simulink library "SIXOSEM_F_STAGE_MASTER_backup20190220"  (Simulink 8.6)
settings: Solver=ode45  StartTime=0.0  StopTime=10.0  RelTol=1e-3
libraries: cdsEpicsOut x52, cdsFilt x31, cdsTP x24, cdsFiltCtrl x9, cdsEpicsIn x9, cdsMuxMatrix x6, VIS_LIB x3, cdsEpicsBinIn x2, lockin x2, SIXOSEM_F_COILOUTF_MASTER x1, rtdemod x1, cdsOsc x1
(part 4 of 5)

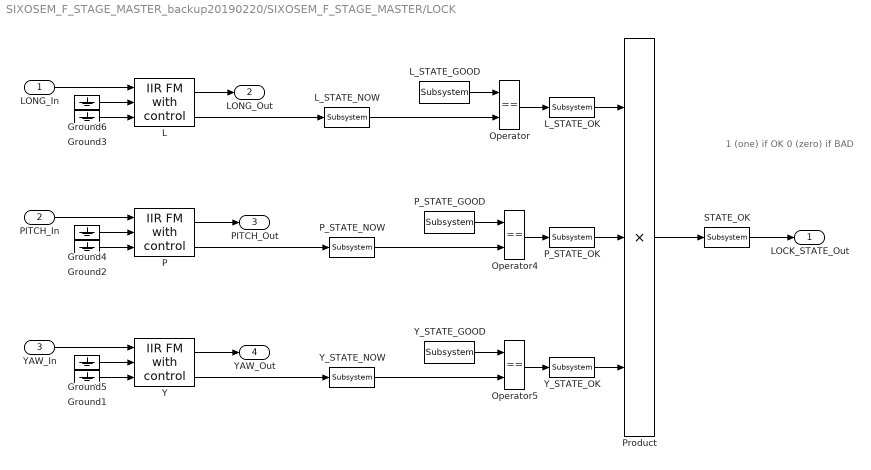
== system SIXOSEM_F_STAGE_MASTER_backup20190220/SIXOSEM_F_STAGE_MASTER/LOCK ==
  note: 1 (one) if OK
      | 0 (zero) if BAD
  LONG_In : Inport
  PITCH_In : Inport  Port=2
  YAW_In : Inport  Port=3
  Ground{1..6} (6 alike) : Ground
  L : cdsFiltCtrl/IIR FM with control  Tag=cdsFiltCtrl  Description=|
      | cdsFiltCntrl is the standard IIR filter module (exactly the same as cdsFilt) but with added control data output 'Ctrl'. Filter module digital signal output appears on the first output, which is called 'Val'. 'Ctrl' output has a bit pattern encoding the state of filter's on/off switches (FM1 through FM10). The bit values are:
      |                                                                                                                                                                                                                                                                                                                                       
      | module 	hex	dec                                                                                                                                                                                                                                                                                                                       
      | -----------------------                                                                                                                                                                                                                                                                                                               
      | FM1	0x20                    32                                                                                                                                                                                                                                                                                                        
      | FM2	0x80                     128                                                                                                                                                                                                                                                                                                      
      | FM3	0x200                   512                                                                                                                                                                                                                                                                                                       
      | FM4	0x800                   2048                                                                                                                                                                                                                                                                                                      
      | FM5	0x2000                 8192                                                                                                                                                                                                                                                                                                       
      | FM6	0x8000                 32768                                                                                                                                                                                                                                                                                                      
      | FM7	0x20000                131072                                                                                                                                                                                                                                                                                                     
      | FM8	0x80000                 524288                                                                                                                                                                                                                                                                                                    
      | FM9	0x200000               2097152                                                                                                                                                                                                                                                                                                    
      | FM10	0x800000               8388608                                                                                                                                                                                                                                                                                                   
      |                                                                                                                                                                                                                                                                                                                                       
      | This bit data can be used to drive some other switches or it can be output using a binary I/O module.
      settings: AttributesFormatString=%<Tag>
  L_STATE_GOOD : cdsEpicsIn/Subsystem  Tag=cdsEpicsIn  Description=|
      | Purpose:                                                                              
      | Create an EPICS input channel connection to the FE realtime controls.                 
      |                                                                                       
      | Operation:                                                                            
      | Outputs value from an EPICS ai record. Value is floating point with a precision of 3..
      |                                                                                       
      | Usage:                                                                                
      | Name the part with the desired EPICS channel name.
      settings: AttributesFormatString=%<Tag>
  L_STATE_NOW : cdsEpicsOut/Subsystem  Tag=cdsEpicsOutput  Description=|
      | Purpose:                                          
      | Output a FE signal to an EPICS channel.           
      |                                                   
      | Operation:                                        
      | Takes input value and passes it to EPICS record.  
      |                                                   
      | Usage:                                            
      | Name the part with the desired EPICS rrecord name.
      settings: AttributesFormatString=%<Tag>
  L_STATE_OK : cdsEpicsOut/Subsystem  Tag=cdsEpicsOutput  Description=|
      | Purpose:                                          
      | Output a FE signal to an EPICS channel.           
      |                                                   
      | Operation:                                        
      | Takes input value and passes it to EPICS record.  
      |                                                   
      | Usage:                                            
      | Name the part with the desired EPICS rrecord name.
      settings: AttributesFormatString=%<Tag>
  Operator : RelationalOperator  Operator===  OutDataTypeStr=boolean
  Operator4 : RelationalOperator  Operator===  OutDataTypeStr=boolean
  Operator5 : RelationalOperator  Operator===  OutDataTypeStr=boolean
  P : cdsFiltCtrl/IIR FM with control  Tag=cdsFiltCtrl  Description=|
      | cdsFiltCntrl is the standard IIR filter module (exactly the same as cdsFilt) but with added control data output 'Ctrl'. Filter module digital signal output appears on the first output, which is called 'Val'. 'Ctrl' output has a bit pattern encoding the state of filter's on/off switches (FM1 through FM10). The bit values are:
      |                                                                                                                                                                                                                                                                                                                                       
      | module 	hex	dec                                                                                                                                                                                                                                                                                                                       
      | -----------------------                                                                                                                                                                                                                                                                                                               
      | FM1	0x20                    32                                                                                                                                                                                                                                                                                                        
      | FM2	0x80                     128                                                                                                                                                                                                                                                                                                      
      | FM3	0x200                   512                                                                                                                                                                                                                                                                                                       
      | FM4	0x800                   2048                                                                                                                                                                                                                                                                                                      
      | FM5	0x2000                 8192                                                                                                                                                                                                                                                                                                       
      | FM6	0x8000                 32768                                                                                                                                                                                                                                                                                                      
      | FM7	0x20000                131072                                                                                                                                                                                                                                                                                                     
      | FM8	0x80000                 524288                                                                                                                                                                                                                                                                                                    
      | FM9	0x200000               2097152                                                                                                                                                                                                                                                                                                    
      | FM10	0x800000               8388608                                                                                                                                                                                                                                                                                                   
      |                                                                                                                                                                                                                                                                                                                                       
      | This bit data can be used to drive some other switches or it can be output using a binary I/O module.
      settings: AttributesFormatString=%<Tag>
  P_STATE_GOOD : cdsEpicsIn/Subsystem  Tag=cdsEpicsIn  Description=|
      | Purpose:                                                                              
      | Create an EPICS input channel connection to the FE realtime controls.                 
      |                                                                                       
      | Operation:                                                                            
      | Outputs value from an EPICS ai record. Value is floating point with a precision of 3..
      |                                                                                       
      | Usage:                                                                                
      | Name the part with the desired EPICS channel name.
      settings: AttributesFormatString=%<Tag>
  P_STATE_NOW : cdsEpicsOut/Subsystem  Tag=cdsEpicsOutput  Description=|
      | Purpose:                                          
      | Output a FE signal to an EPICS channel.           
      |                                                   
      | Operation:                                        
      | Takes input value and passes it to EPICS record.  
      |                                                   
      | Usage:                                            
      | Name the part with the desired EPICS rrecord name.
      settings: AttributesFormatString=%<Tag>
  P_STATE_OK : cdsEpicsOut/Subsystem  Tag=cdsEpicsOutput  Description=|
      | Purpose:                                          
      | Output a FE signal to an EPICS channel.           
      |                                                   
      | Operation:                                        
      | Takes input value and passes it to EPICS record.  
      |                                                   
      | Usage:                                            
      | Name the part with the desired EPICS rrecord name.
      settings: AttributesFormatString=%<Tag>
  Product : Product  Inputs=3  RndMeth=Zero
  STATE_OK : cdsEpicsOut/Subsystem  Tag=cdsEpicsOutput  Description=|
      | Purpose:                                          
      | Output a FE signal to an EPICS channel.           
      |                                                   
      | Operation:                                        
      | Takes input value and passes it to EPICS record.  
      |                                                   
      | Usage:                                            
      | Name the part with the desired EPICS rrecord name.
      settings: AttributesFormatString=%<Tag>
  Y : cdsFiltCtrl/IIR FM with control  Tag=cdsFiltCtrl  Description=|
      | cdsFiltCntrl is the standard IIR filter module (exactly the same as cdsFilt) but with added control data output 'Ctrl'. Filter module digital signal output appears on the first output, which is called 'Val'. 'Ctrl' output has a bit pattern encoding the state of filter's on/off switches (FM1 through FM10). The bit values are:
      |                                                                                                                                                                                                                                                                                                                                       
      | module 	hex	dec                                                                                                                                                                                                                                                                                                                       
      | -----------------------                                                                                                                                                                                                                                                                                                               
      | FM1	0x20                    32                                                                                                                                                                                                                                                                                                        
      | FM2	0x80                     128                                                                                                                                                                                                                                                                                                      
      | FM3	0x200                   512                                                                                                                                                                                                                                                                                                       
      | FM4	0x800                   2048                                                                                                                                                                                                                                                                                                      
      | FM5	0x2000                 8192                                                                                                                                                                                                                                                                                                       
      | FM6	0x8000                 32768                                                                                                                                                                                                                                                                                                      
      | FM7	0x20000                131072                                                                                                                                                                                                                                                                                                     
      | FM8	0x80000                 524288                                                                                                                                                                                                                                                                                                    
      | FM9	0x200000               2097152                                                                                                                                                                                                                                                                                                    
      | FM10	0x800000               8388608                                                                                                                                                                                                                                                                                                   
      |                                                                                                                                                                                                                                                                                                                                       
      | This bit data can be used to drive some other switches or it can be output using a binary I/O module.
      settings: AttributesFormatString=%<Tag>
  Y_STATE_GOOD : cdsEpicsIn/Subsystem  Tag=cdsEpicsIn  Description=|
      | Purpose:                                                                              
      | Create an EPICS input channel connection to the FE realtime controls.                 
      |                                                                                       
      | Operation:                                                                            
      | Outputs value from an EPICS ai record. Value is floating point with a precision of 3..
      |                                                                                       
      | Usage:                                                                                
      | Name the part with the desired EPICS channel name.
      settings: AttributesFormatString=%<Tag>
  Y_STATE_NOW : cdsEpicsOut/Subsystem  Tag=cdsEpicsOutput  Description=|
      | Purpose:                                          
      | Output a FE signal to an EPICS channel.           
      |                                                   
      | Operation:                                        
      | Takes input value and passes it to EPICS record.  
      |                                                   
      | Usage:                                            
      | Name the part with the desired EPICS rrecord name.
      settings: AttributesFormatString=%<Tag>
  Y_STATE_OK : cdsEpicsOut/Subsystem  Tag=cdsEpicsOutput  Description=|
      | Purpose:                                          
      | Output a FE signal to an EPICS channel.           
      |                                                   
      | Operation:                                        
      | Takes input value and passes it to EPICS record.  
      |                                                   
      | Usage:                                            
      | Name the part with the desired EPICS rrecord name.
      settings: AttributesFormatString=%<Tag>
  LOCK_STATE_Out : Outport
  LONG_Out : Outport  Port=2
  PITCH_Out : Outport  Port=3
  YAW_Out : Outport  Port=4
  wires:
  Ground6/1 -> L/2
  L_STATE_GOOD/1 -> Operator/1
  L/2 -> L_STATE_NOW/1
  L/1 -> LONG_Out/1
  LONG_In/1 -> L/1
  P/1 -> PITCH_Out/1
  Ground4/1 -> P/2
  PITCH_In/1 -> P/1
  P_STATE_GOOD/1 -> Operator4/1
  P/2 -> P_STATE_NOW/1
  Ground5/1 -> Y/2
  YAW_In/1 -> Y/1
  Y_STATE_GOOD/1 -> Operator5/1
  Y/2 -> Y_STATE_NOW/1
  Y/1 -> YAW_Out/1
  Operator/1 -> L_STATE_OK/1
  Operator4/1 -> P_STATE_OK/1
  Operator5/1 -> Y_STATE_OK/1
  Product/1 -> STATE_OK/1
  P_STATE_OK/1 -> Product/2
  L_STATE_OK/1 -> Product/1
  Y_STATE_OK/1 -> Product/3
  STATE_OK/1 -> LOCK_STATE_Out/1
  L_STATE_NOW/1 -> Operator/2
  Y_STATE_NOW/1 -> Operator5/2
  P_STATE_NOW/1 -> Operator4/2
  Ground1/1 -> Y/3
  Ground2/1 -> P/3
  Ground3/1 -> L/3

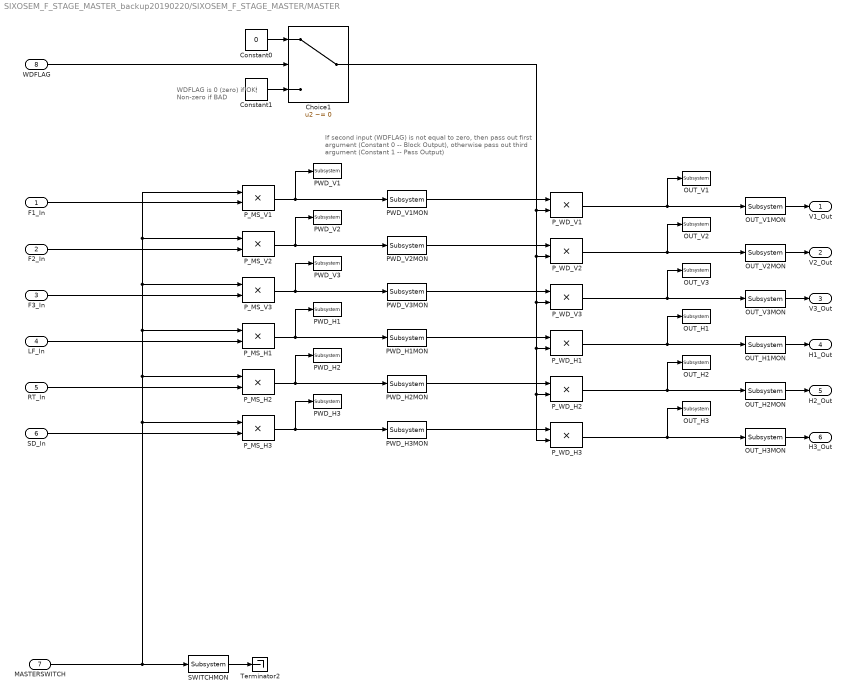
== system SIXOSEM_F_STAGE_MASTER_backup20190220/SIXOSEM_F_STAGE_MASTER/MASTER ==
  note: WDFLAG is 0 (zero) if OK,
      | Non-zero if BAD
  note: If second input (WDFLAG) is not equal to zero,
      | then pass out first argument (Constant 0 -- Block Output),
      | otherwise pass out third argument (Constant 1 -- Pass Output)
  F1_In : Inport
  F2_In : Inport  Port=2
  F3_In : Inport  Port=3
  LF_In : Inport  Port=4
  RT_In : Inport  Port=5
  SD_In : Inport  Port=6
  MASTERSWITCH : Inport  Port=7
  WDFLAG : Inport  Port=8
  Choice1 : Switch  Criteria=u2 ~= 0  Threshold=0.5
  Constant0 : Constant  Value=0
  Constant1 : Constant
  OUT_H1 : cdsTP/Subsystem  Tag=Test Point
      settings: AttributesFormatString=%<Tag>
  OUT_H1MON : cdsEpicsOut/Subsystem  Tag=cdsEpicsOutput  Description=|
      | Purpose:                                          
      | Output a FE signal to an EPICS channel.           
      |                                                   
      | Operation:                                        
      | Takes input value and passes it to EPICS record.  
      |                                                   
      | Usage:                                            
      | Name the part with the desired EPICS rrecord name.
      settings: AttributesFormatString=%<Tag>
  OUT_H2 : cdsTP/Subsystem  Tag=Test Point
      settings: AttributesFormatString=%<Tag>
  OUT_H2MON : cdsEpicsOut/Subsystem  Tag=cdsEpicsOutput  Description=|
      | Purpose:                                          
      | Output a FE signal to an EPICS channel.           
      |                                                   
      | Operation:                                        
      | Takes input value and passes it to EPICS record.  
      |                                                   
      | Usage:                                            
      | Name the part with the desired EPICS rrecord name.
      settings: AttributesFormatString=%<Tag>
  OUT_H3 : cdsTP/Subsystem  Tag=Test Point
      settings: AttributesFormatString=%<Tag>
  OUT_H3MON : cdsEpicsOut/Subsystem  Tag=cdsEpicsOutput  Description=|
      | Purpose:                                          
      | Output a FE signal to an EPICS channel.           
      |                                                   
      | Operation:                                        
      | Takes input value and passes it to EPICS record.  
      |                                                   
      | Usage:                                            
      | Name the part with the desired EPICS rrecord name.
      settings: AttributesFormatString=%<Tag>
  OUT_V1 : cdsTP/Subsystem  Tag=Test Point
      settings: AttributesFormatString=%<Tag>
  OUT_V1MON : cdsEpicsOut/Subsystem  Tag=cdsEpicsOutput  Description=|
      | Purpose:                                          
      | Output a FE signal to an EPICS channel.           
      |                                                   
      | Operation:                                        
      | Takes input value and passes it to EPICS record.  
      |                                                   
      | Usage:                                            
      | Name the part with the desired EPICS rrecord name.
      settings: AttributesFormatString=%<Tag>
  OUT_V2 : cdsTP/Subsystem  Tag=Test Point
      settings: AttributesFormatString=%<Tag>
  OUT_V2MON : cdsEpicsOut/Subsystem  Tag=cdsEpicsOutput  Description=|
      | Purpose:                                          
      | Output a FE signal to an EPICS channel.           
      |                                                   
      | Operation:                                        
      | Takes input value and passes it to EPICS record.  
      |                                                   
      | Usage:                                            
      | Name the part with the desired EPICS rrecord name.
      settings: AttributesFormatString=%<Tag>
  OUT_V3 : cdsTP/Subsystem  Tag=Test Point
      settings: AttributesFormatString=%<Tag>
  OUT_V3MON : cdsEpicsOut/Subsystem  Tag=cdsEpicsOutput  Description=|
      | Purpose:                                          
      | Output a FE signal to an EPICS channel.           
      |                                                   
      | Operation:                                        
      | Takes input value and passes it to EPICS record.  
      |                                                   
      | Usage:                                            
      | Name the part with the desired EPICS rrecord name.
      settings: AttributesFormatString=%<Tag>
  PWD_H1 : cdsTP/Subsystem  Tag=Test Point
      settings: AttributesFormatString=%<Tag>
  PWD_H1MON : cdsEpicsOut/Subsystem  Tag=cdsEpicsOutput  Description=|
      | Purpose:                                          
      | Output a FE signal to an EPICS channel.           
      |                                                   
      | Operation:                                        
      | Takes input value and passes it to EPICS record.  
      |                                                   
      | Usage:                                            
      | Name the part with the desired EPICS rrecord name.
      settings: AttributesFormatString=%<Tag>
  PWD_H2 : cdsTP/Subsystem  Tag=Test Point
      settings: AttributesFormatString=%<Tag>
  PWD_H2MON : cdsEpicsOut/Subsystem  Tag=cdsEpicsOutput  Description=|
      | Purpose:                                          
      | Output a FE signal to an EPICS channel.           
      |                                                   
      | Operation:                                        
      | Takes input value and passes it to EPICS record.  
      |                                                   
      | Usage:                                            
      | Name the part with the desired EPICS rrecord name.
      settings: AttributesFormatString=%<Tag>
  PWD_H3 : cdsTP/Subsystem  Tag=Test Point
      settings: AttributesFormatString=%<Tag>
  PWD_H3MON : cdsEpicsOut/Subsystem  Tag=cdsEpicsOutput  Description=|
      | Purpose:                                          
      | Output a FE signal to an EPICS channel.           
      |                                                   
      | Operation:                                        
      | Takes input value and passes it to EPICS record.  
      |                                                   
      | Usage:                                            
      | Name the part with the desired EPICS rrecord name.
      settings: AttributesFormatString=%<Tag>
  PWD_V1 : cdsTP/Subsystem  Tag=Test Point
      settings: AttributesFormatString=%<Tag>
  PWD_V1MON : cdsEpicsOut/Subsystem  Tag=cdsEpicsOutput  Description=|
      | Purpose:                                          
      | Output a FE signal to an EPICS channel.           
      |                                                   
      | Operation:                                        
      | Takes input value and passes it to EPICS record.  
      |                                                   
      | Usage:                                            
      | Name the part with the desired EPICS rrecord name.
      settings: AttributesFormatString=%<Tag>
  PWD_V2 : cdsTP/Subsystem  Tag=Test Point
      settings: AttributesFormatString=%<Tag>
  PWD_V2MON : cdsEpicsOut/Subsystem  Tag=cdsEpicsOutput  Description=|
      | Purpose:                                          
      | Output a FE signal to an EPICS channel.           
      |                                                   
      | Operation:                                        
      | Takes input value and passes it to EPICS record.  
      |                                                   
      | Usage:                                            
      | Name the part with the desired EPICS rrecord name.
      settings: AttributesFormatString=%<Tag>
  PWD_V3 : cdsTP/Subsystem  Tag=Test Point
      settings: AttributesFormatString=%<Tag>
  PWD_V3MON : cdsEpicsOut/Subsystem  Tag=cdsEpicsOutput  Description=|
      | Purpose:                                          
      | Output a FE signal to an EPICS channel.           
      |                                                   
      | Operation:                                        
      | Takes input value and passes it to EPICS record.  
      |                                                   
      | Usage:                                            
      | Name the part with the desired EPICS rrecord name.
      settings: AttributesFormatString=%<Tag>
  P_MS_H1 : Product  RndMeth=Zero
  P_MS_H2 : Product  RndMeth=Zero
  P_MS_H3 : Product  RndMeth=Zero
  P_MS_V1 : Product  RndMeth=Zero
  P_MS_V2 : Product  RndMeth=Zero
  P_MS_V3 : Product  RndMeth=Zero
  P_WD_H1 : Product  RndMeth=Zero
  P_WD_H2 : Product  RndMeth=Zero
  P_WD_H3 : Product  RndMeth=Zero
  P_WD_V1 : Product  RndMeth=Zero
  P_WD_V2 : Product  RndMeth=Zero
  P_WD_V3 : Product  RndMeth=Zero
  SWITCHMON : cdsEpicsOut/Subsystem  Tag=cdsEpicsOutput  Description=|
      | Purpose:                                          
      | Output a FE signal to an EPICS channel.           
      |                                                   
      | Operation:                                        
      | Takes input value and passes it to EPICS record.  
      |                                                   
      | Usage:                                            
      | Name the part with the desired EPICS rrecord name.
      settings: AttributesFormatString=%<Tag>
  Terminator2 : Terminator
  V1_Out : Outport
  V2_Out : Outport  Port=2
  V3_Out : Outport  Port=3
  H1_Out : Outport  Port=4
  H2_Out : Outport  Port=5
  H3_Out : Outport  Port=6
  wires:
  Choice1/1 -> P_WD_V1/2, P_WD_V2/2, P_WD_V3/2, P_WD_H1/2, P_WD_H2/2, P_WD_H3/2
  PWD_H3MON/1 -> P_WD_H3/1
  PWD_H2MON/1 -> P_WD_H2/1
  PWD_H1MON/1 -> P_WD_H1/1
  PWD_V3MON/1 -> P_WD_V3/1
  PWD_V2MON/1 -> P_WD_V2/1
  PWD_V1MON/1 -> P_WD_V1/1
  WDFLAG/1 -> Choice1/2
  Constant0/1 -> Choice1/1
  Constant1/1 -> Choice1/3
  P_WD_H3/1 -> OUT_H3/1, OUT_H3MON/1
  P_WD_H2/1 -> OUT_H2/1, OUT_H2MON/1
  P_WD_H1/1 -> OUT_H1/1, OUT_H1MON/1
  P_WD_V3/1 -> OUT_V3/1, OUT_V3MON/1
  P_WD_V2/1 -> OUT_V2/1, OUT_V2MON/1
  P_WD_V1/1 -> OUT_V1/1, OUT_V1MON/1
  P_MS_H3/1 -> PWD_H3MON/1, PWD_H3/1
  P_MS_H2/1 -> PWD_H2MON/1, PWD_H2/1
  P_MS_H1/1 -> PWD_H1MON/1, PWD_H1/1
  P_MS_V3/1 -> PWD_V3MON/1, PWD_V3/1
  P_MS_V2/1 -> PWD_V2MON/1, PWD_V2/1
  P_MS_V1/1 -> PWD_V1MON/1, PWD_V1/1
  OUT_H2MON/1 -> H2_Out/1
  OUT_H3MON/1 -> H3_Out/1
  OUT_H1MON/1 -> H1_Out/1
  OUT_V3MON/1 -> V3_Out/1
  OUT_V1MON/1 -> V1_Out/1
  OUT_V2MON/1 -> V2_Out/1
  MASTERSWITCH/1 -> P_MS_H3/1, P_MS_H2/1, P_MS_H1/1, P_MS_V3/1, P_MS_V2/1, P_MS_V1/1, SWITCHMON/1
  SD_In/1 -> P_MS_H3/2
  RT_In/1 -> P_MS_H2/2
  LF_In/1 -> P_MS_H1/2
  F3_In/1 -> P_MS_V3/2
  F2_In/1 -> P_MS_V2/2
  F1_In/1 -> P_MS_V1/2
  SWITCHMON/1 -> Terminator2/1

== system SIXOSEM_F_STAGE_MASTER_backup20190220/SIXOSEM_F_STAGE_MASTER/OPTICALIGN ==
  Ground1 : Ground
  Ground2 : Ground
  P : cdsFilt/Subsystem  Tag=cdsFilt  Description=|
      | Purpose:                                                                                                                                                                                                                                  
      | Standard CDS IIR filter module.                                                                                                                                                                                                           
      |                                                                                                                                                                                                                                           
      | Operation:                                                                                                                                                                                                                                
      | Consists of 10 second order section IIR filters, plus a ramped gain stage. In FE code, also provides pre-defined test points and excitation channel inputs. The filter coefficients are defined in the LIGO system using the 'foton' tool.
      |                                                                                                                                                                                                                                           
      | Usage:                                                                                                                                                                                                                                    
      | Name the part with the desired filter module name.
      settings: AttributesFormatString=%<Tag>
  Y : cdsFilt/Subsystem  Tag=cdsFilt  Description=|
      | Purpose:                                                                                                                                                                                                                                  
      | Standard CDS IIR filter module.                                                                                                                                                                                                           
      |                                                                                                                                                                                                                                           
      | Operation:                                                                                                                                                                                                                                
      | Consists of 10 second order section IIR filters, plus a ramped gain stage. In FE code, also provides pre-defined test points and excitation channel inputs. The filter coefficients are defined in the LIGO system using the 'foton' tool.
      |                                                                                                                                                                                                                                           
      | Usage:                                                                                                                                                                                                                                    
      | Name the part with the desired filter module name.
      settings: AttributesFormatString=%<Tag>
  PITCH_Out : Outport
  YAW_Out : Outport  Port=2
  wires:
  Ground2/1 -> Y/1
  Ground1/1 -> P/1
  P/1 -> PITCH_Out/1
  Y/1 -> YAW_Out/1
